simulink model "ssc_p"  (R2017b)
settings: Solver=ode45  StartTime=0.0  StopTime=10.0  RelTol=1e-3  EnableMultiTasking=on
settings Model: Creator=user  LastModifiedBy=c.chawla
settings SolverCC: ZeroCrossAlgorithm=Adaptive
settings DataIOCC: LimitDataPoints=on  SaveFormat=Array
settings OptimizationCC: LifeSpan=inf  SimCompilerOptimization=on
settings DebuggingCC: UnderspecifiedInitializationDetection=Classic  MergeDetectMultiDrivingBlocksExec=none  SFUnexpectedBacktrackingDiag=warning  SFNoUnconditionalDefaultTransitionDiag=warning  SFExecutionAtInitializationDiag=none
settings HardwareCC: ProdBitPerPointer=32  ProdBitPerSizeT=32  ProdBitPerPtrDiffT=32  ProdLargestAtomicFloat=None  ProdIntDivRoundTo=Undefined  ProdEndianess=Unspecified  ProdWordSize=32  ProdHWDeviceType=32-bit Generic
settings ModelReferenceCC: PropagateSignalLabelsOutOfModel=off
settings CodeAppCC: StateflowObjectComments=on
settings GRTTargetCC: TargetLangStandard=C89/C90 (ANSI)  GeneratePreprocessorConditionals=Disable all
settings ConfigComp: CovMetricSettings=dw  CovHtmlReporting=on  CovSaveCumulativeToWorkspaceVar=on  CovSaveSingleToWorkspaceVar=on  CovExternalEMLEnable=off  CovSFcnEnable=off
settings ConfigurationSet: Description=SimMechanics 2G

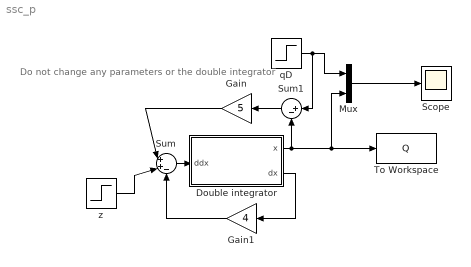
== system ssc_p ==
  note: Do not change any parameters or the double integrator
  Double integrator : Subsystem
      mask Display: dpoly([1],[1 0 0], 's')
  Gain : Gain  Gain=5
  Gain1 : Gain  Gain=4
  Mux : Mux  Inputs=2
  Scope : Scope
  Sum : Sum  Inputs=|++-
  Sum1 : Sum  Inputs=|+-
  To Workspace : ToWorkspace  VariableName=Q  SaveFormat=Timeseries  SampleTime=-1
  qD : Step  Time=0  After=pi/2  SampleTime=0
  z : Step  Time=0  After=0.3  SampleTime=0
  wires:
  Gain/1 -> Sum/1
  Double integrator/2(dx) -> Gain1/1
  Gain1/1 -> Sum/3
  Sum/1 -> Double integrator/1(ddx)
  z/1 -> Sum/2
  Double integrator/1(x) -> Sum1/2, Mux/2, To Workspace/1
  qD/1 -> Sum1/1, Mux/1
  Mux/1 -> Scope/1
  Sum1/1 -> Gain/1

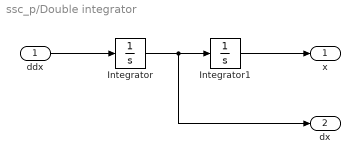
== system ssc_p/Double integrator ==
  ddx : Inport
  Integrator : Integrator
  Integrator1 : Integrator
  x : Outport
  dx : Outport  Port=2
  wires:
  Integrator/1 -> dx/1, Integrator1/1
  Integrator1/1 -> x/1
  ddx/1 -> Integrator/1
